simulink model "causality_av_s"  (R2021b)
settings: Solver=VariableStepAuto  StartTime=0.0  StopTime=10.0  RelTol=1e-3
values from neighbouring files (symbols this model uses):
  battery =     [matlab.mat]
  car =     [matlab.mat]
  environment =     [matlab.mat]
  lidar =     [matlab.mat]
  pedestrian =     [matlab.mat]
settings Model: Creator=hugol  LastModifiedBy=hugoaraujo
settings SolverCC: AlgebraicLoopSolver=TrustRegion
settings DataIOCC: ReturnWorkspaceOutputs=off
settings DebuggingCC: SFMachineParentedDataDiag=warning  ArithmeticOperatorsInVariantConditions=warning
settings SFSimCC: CustomCodeUndefinedFunction=UseInterfaceOnly

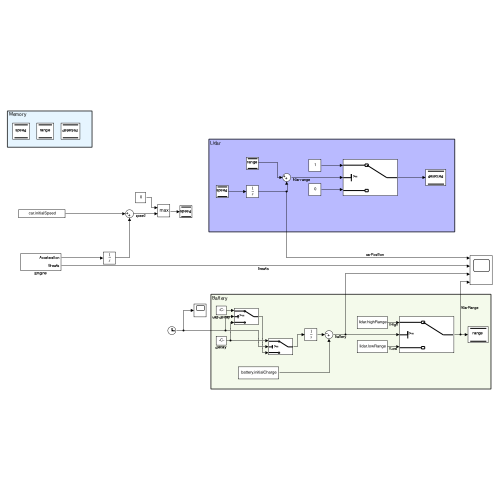
[thumbnail: Simulink's stored preview of the top-level diagram]
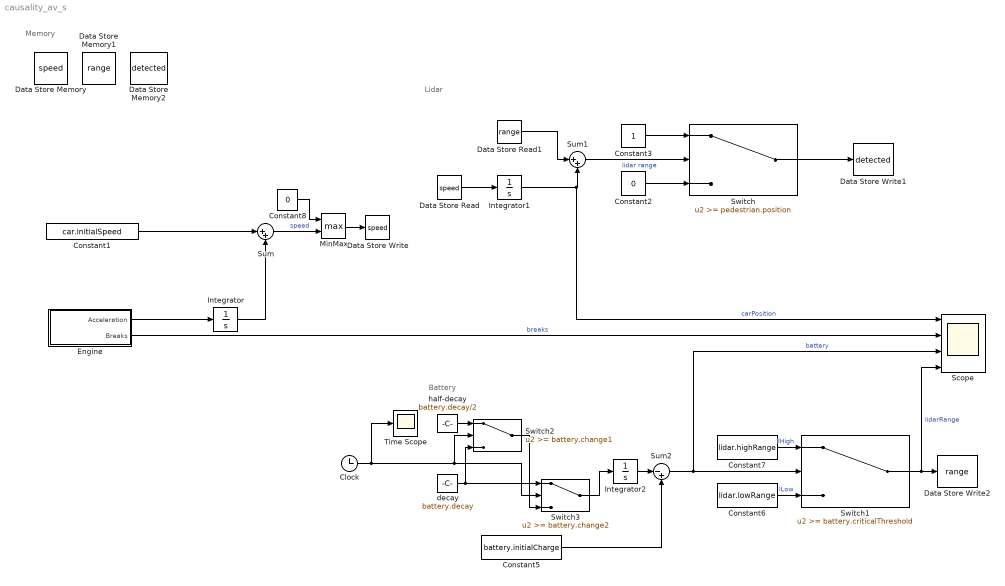
== system causality_av_s ==
  note: Lidar
  note: Memory
  note: Battery
  Clock : Clock
  Constant1 : Constant  Value=car.initialSpeed
  Constant2 : Constant  Value=0
  Constant3 : Constant
  Constant5 : Constant  Value=battery.initialCharge
  Constant6 : Constant  Value=lidar.lowRange
  Constant7 : Constant  Value=lidar.highRange
  Constant8 : Constant  Value=0
  Data Store Memory : DataStoreMemory  DataStoreName=speed  ReadBeforeWriteMsg=warning  WriteAfterWriteMsg=warning  WriteAfterReadMsg=warning  ShowAdditionalParam=off
  Data Store Memory1 : DataStoreMemory  DataStoreName=range  ReadBeforeWriteMsg=warning  WriteAfterWriteMsg=warning  WriteAfterReadMsg=warning  ShowAdditionalParam=off
  Data Store Memory2 : DataStoreMemory  DataStoreName=detected  ReadBeforeWriteMsg=warning  WriteAfterWriteMsg=warning  WriteAfterReadMsg=warning  ShowAdditionalParam=off
  Data Store Read : DataStoreRead  DataStoreName=speed  IndexOptions=Index vector (dialog)  Indices=1  OutputSizes=1
  Data Store Read1 : DataStoreRead  DataStoreName=range  IndexOptions=Index vector (dialog)  Indices=1  OutputSizes=1
  Data Store Write : DataStoreWrite  DataStoreName=speed  IndexOptions=Index vector (dialog)  Indices=1  OutputSizes=1
  Data Store Write1 : DataStoreWrite  DataStoreName=detected  IndexOptions=Index vector (dialog)  Indices=1  OutputSizes=1
  Data Store Write2 : DataStoreWrite  DataStoreName=range  IndexOptions=Index vector (dialog)  Indices=1  OutputSizes=1
  Engine : Subsystem
  Integrator : Integrator
  Integrator1 : Integrator
  Integrator2 : Integrator
  MinMax : MinMax  Function=max  Inputs=2
  Scope : Scope  NumInputPorts=4
  Sum : Sum  Inputs=|++
  Sum1 : Sum  Inputs=|++
  Sum2 : Sum  Inputs=|-+
  Switch : Switch  Threshold=pedestrian.position
  Switch1 : Switch  Threshold=battery.criticalThreshold
  Switch2 : Switch  Threshold=battery.change1
  Switch3 : Switch  Threshold=battery.change2
  Time Scope : Scope
  decay : Constant  Value=battery.decay
  half-decay : Constant  Value=battery.decay/2
  wires:
  Constant1/1 -> Sum/1
  Integrator/1 -> Sum/2
  Integrator1/1 -> Scope/1, Sum1/2  "carPosition"
  Data Store Read1/1 -> Sum1/1
  Switch/1 -> Data Store Write1/1
  Sum1/1 -> Switch/2  "lidar range"
  Constant2/1 -> Switch/3
  Constant3/1 -> Switch/1
  Engine/1(Acceleration) -> Integrator/1
  Data Store Read/1 -> Integrator1/1
  Constant5/1 -> Sum2/2
  Integrator2/1 -> Sum2/1
  Sum2/1 -> Scope/3, Switch1/2  "battery"
  Constant7/1 -> Switch1/1  "lHigh"
  Switch1/1 -> Scope/4, Data Store Write2/1  "lidarRange"
  MinMax/1 -> Data Store Write/1
  Sum/1 -> MinMax/2  "speed"
  Constant8/1 -> MinMax/1
  Engine/2(Breaks) -> Scope/2  "breaks"
  Constant6/1 -> Switch1/3  "lLow"
  Clock/1 -> Switch3/2, Switch2/2, Time Scope/1
  decay/1 -> Switch3/1, Switch2/3
  half-decay/1 -> Switch2/1
  Switch3/1 -> Integrator2/1
  Switch2/1 -> Switch3/3

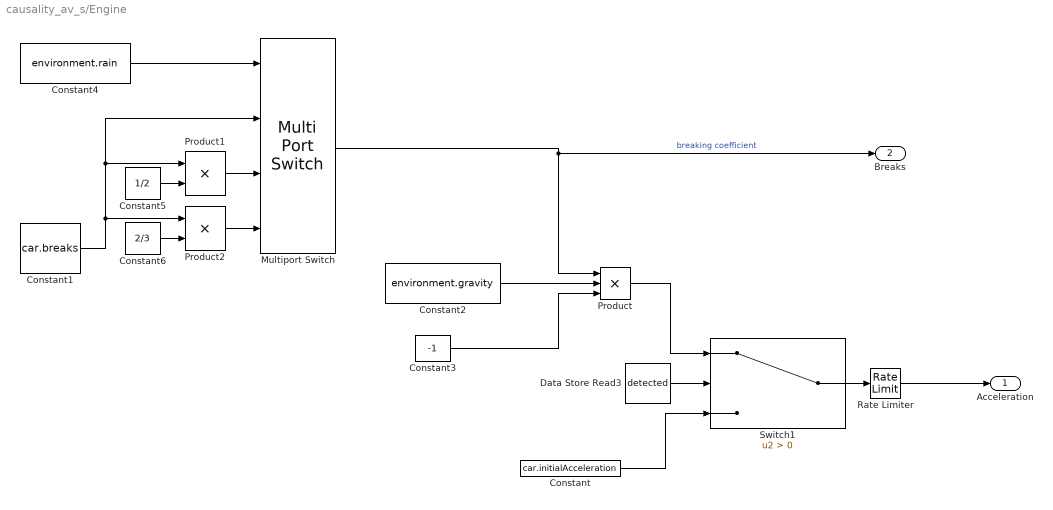
== system causality_av_s/Engine ==
  Constant : Constant  Value=car.initialAcceleration
  Constant1 : Constant  Value=car.breaks
  Constant2 : Constant  Value=environment.gravity
  Constant3 : Constant  Value=-1
  Constant4 : Constant  Value=environment.rain
  Constant5 : Constant  Value=1/2
  Constant6 : Constant  Value=2/3
  Data Store Read3 : DataStoreRead  DataStoreName=detected  IndexOptions=Index vector (dialog)  Indices=1  OutputSizes=1
  Multiport Switch : MultiPortSwitch  DataPortOrder=Zero-based contiguous  zeroidx=on
  Product : Product  Inputs=3
  Product1 : Product
  Product2 : Product
  Rate Limiter : RateLimiter  RisingSlewLimit=10  FallingSlewLimit=-10  SampleTimeMode=inherited
  Switch1 : Switch  Criteria=u2 > Threshold
  Acceleration : Outport  VectorParamsAs1DForOutWhenUnconnected=off
  Breaks : Outport  Port=2  VectorParamsAs1DForOutWhenUnconnected=off
  wires:
  Data Store Read3/1 -> Switch1/2
  Constant/1 -> Switch1/3
  Constant2/1 -> Product/2
  Constant3/1 -> Product/3
  Product/1 -> Switch1/1
  Switch1/1 -> Rate Limiter/1
  Constant4/1 -> Multiport Switch/1
  Constant1/1 -> Multiport Switch/2, Product1/1, Product2/1
  Product1/1 -> Multiport Switch/3
  Product2/1 -> Multiport Switch/4
  Constant5/1 -> Product1/2
  Constant6/1 -> Product2/2
  Multiport Switch/1 -> Breaks/1, Product/1  "breaking coefficient"
  Rate Limiter/1 -> Acceleration/1
